simulink model "M14"  (R2018a)
settings: Solver=VariableStepAuto  StartTime=0.0  StopTime=6  RelTol=1e-3
settings Model: Creator=admin  LastModifiedBy=admin

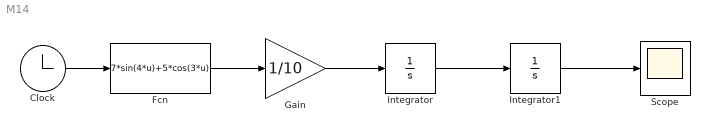
== system M14 ==
  Clock : Clock
  Fcn : Fcn  Expr=7*sin(4*u)+5*cos(3*u)
  Gain : Gain  Gain=1/10
  Integrator : Integrator  InitialCondition=1
  Integrator1 : Integrator  InitialCondition=4
  Scope : Scope
  wires:
  Clock/1 -> Fcn/1
  Integrator/1 -> Integrator1/1
  Fcn/1 -> Gain/1
  Gain/1 -> Integrator/1
  Integrator1/1 -> Scope/1
